simulink model "l5MV"  (R2024a)
settings: Solver=VariableStepAuto  StartTime=0.0  StopTime=200  RelTol=1e-3
settings Model: Creator=sprinkle  LastModifiedBy=ZY395
settings OptimizationCC: ReuseModelBlockBuffer=off
settings RTWCC: GPUComputeCapability=3.5

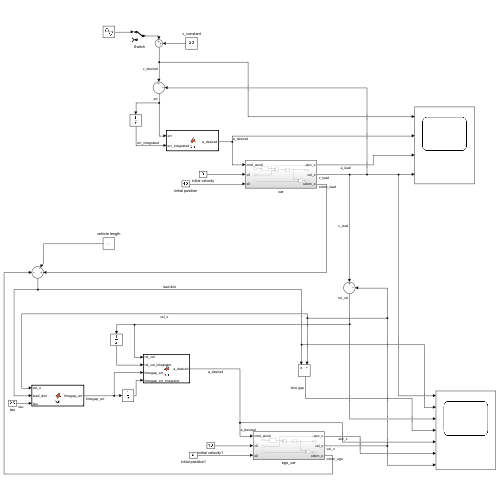
[thumbnail: Simulink's stored preview of the top-level diagram]
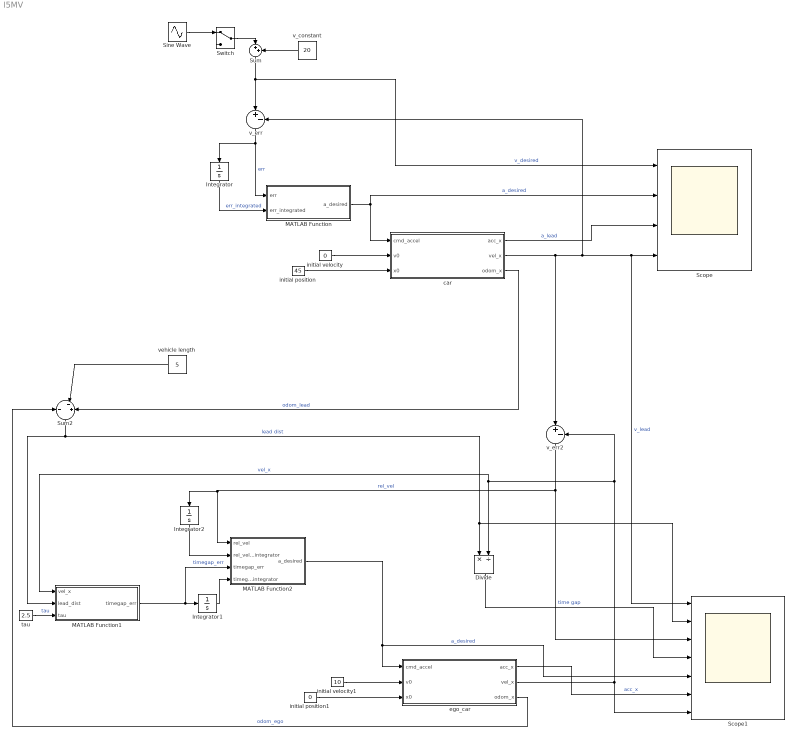
== system l5MV ==
  Divide : Product  Inputs=*/
  Integrator : Integrator
  Integrator1 : Integrator
  Integrator2 : Integrator
  MATLAB Function : MATLAB Function  TreatAsAtomicUnit=on
  MATLAB Function1 : MATLAB Function  TreatAsAtomicUnit=on
  MATLAB Function2 : MATLAB Function  TreatAsAtomicUnit=on
  Scope : Scope  NumInputPorts=4
  Scope1 : Scope  NumInputPorts=7
  Sine Wave : Sin  Amplitude=5  SampleTime=0
  Sum : Sum  Inputs=|++
  Sum2 : Sum  Inputs=-|-+
  Switch : ManualSwitch
  car : Subsystem
  ego_car : Subsystem
  initial position : Constant  Value=45
  initial position1 : Constant  Value=0
  initial velocity : Constant  Value=0
  initial velocity1 : Constant  Value=10
  tau : Constant  Value=2.5
  v_constant : Constant  Value=20
  v_err : Sum  Inputs=|+-
  v_err2 : Sum  Inputs=|+-
  vehicle length : Constant  Value=5
  wires:
  Integrator2/1 -> MATLAB Function2/2(rel_vel_integrator)
  MATLAB Function1/1(timegap_err) -> MATLAB Function2/3(timegap_err), Integrator1/1  "timegap_err"
  ego_car/2(vel_x) -> Scope1/7, Divide/2, MATLAB Function1/1(vel_x), v_err2/2  "vel_x"
  ego_car/1(acc_x) -> Scope1/6  "acc_x"
  MATLAB Function2/1(a_desired) -> ego_car/1(cmd_accel), Scope1/5  "a_desired"
  tau/1 -> MATLAB Function1/3(tau)  "tau"
  v_err2/1 -> Scope1/3, Integrator2/1, MATLAB Function2/1(rel_vel)  "rel_vel"
  MATLAB Function/1(a_desired) -> Scope/2, car/1(cmd_accel)  "a_desired"
  initial velocity1/1 -> ego_car/2(v0)
  ego_car/3(odom_x) -> Sum2/1  "odom_ego"
  Integrator1/1 -> MATLAB Function2/4(timegap_err_integrator)
  Switch/1 -> Sum/1
  vehicle length/1 -> Sum2/2
  Sine Wave/1 -> Switch/1
  Sum/1 -> Scope/1, v_err/1  "v_desired"
  car/3(odom_x) -> Sum2/3  "odom_lead"
  v_constant/1 -> Sum/2
  Sum2/1 -> MATLAB Function1/2(lead_dist), Scope1/2, Divide/1  "lead dist"
  car/2(vel_x) -> v_err/2, Scope1/1, Scope/4, v_err2/1  "v_lead"
  Integrator/1 -> MATLAB Function/2(err_integrated)  "err_integrated"
  Divide/1 -> Scope1/4  "time gap"
  v_err/1 -> MATLAB Function/1(err), Integrator/1  "err"
  initial position/1 -> car/3(x0)
  car/1(acc_x) -> Scope/3  "a_lead"
  initial velocity/1 -> car/2(v0)
  initial position1/1 -> ego_car/3(x0)

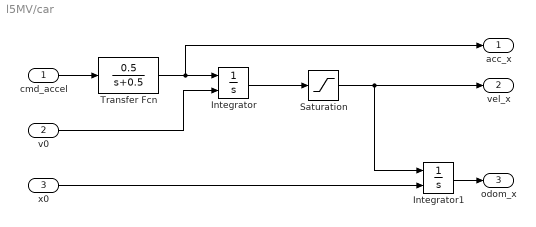
== system l5MV/car ==
  cmd_accel : Inport
  v0 : Inport  Port=2
  x0 : Inport  Port=3
  Integrator : Integrator  InitialConditionSource=external
  Integrator1 : Integrator  InitialConditionSource=external
  Saturation : Saturate  UpperLimit=80  LowerLimit=0
  Transfer Fcn : TransferFcn  Numerator=[0.5]  Denominator=[1 0.5]
  acc_x : Outport
  vel_x : Outport  Port=2
  odom_x : Outport  Port=3
  wires:
  v0/1 -> Integrator/2
  cmd_accel/1 -> Transfer Fcn/1
  Transfer Fcn/1 -> acc_x/1, Integrator/1
  Integrator1/1 -> odom_x/1
  Integrator/1 -> Saturation/1
  x0/1 -> Integrator1/2
  Saturation/1 -> vel_x/1, Integrator1/1

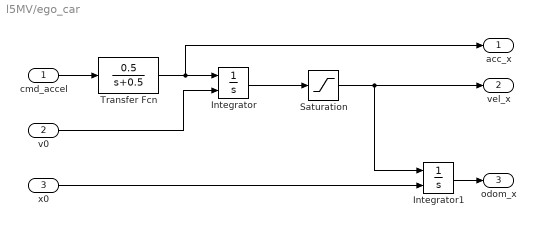
== system l5MV/ego_car ==
  cmd_accel : Inport
  v0 : Inport  Port=2
  x0 : Inport  Port=3
  Integrator : Integrator  InitialConditionSource=external
  Integrator1 : Integrator  InitialConditionSource=external
  Saturation : Saturate  UpperLimit=80  LowerLimit=0
  Transfer Fcn : TransferFcn  Numerator=[0.5]  Denominator=[1 0.5]
  acc_x : Outport
  vel_x : Outport  Port=2
  odom_x : Outport  Port=3
  wires:
  Saturation/1 -> Integrator1/1, vel_x/1
  x0/1 -> Integrator1/2
  Integrator/1 -> Saturation/1
  Integrator1/1 -> odom_x/1
  Transfer Fcn/1 -> Integrator/1, acc_x/1
  cmd_accel/1 -> Transfer Fcn/1
  v0/1 -> Integrator/2

== matlab function l5MV/MATLAB Function1 ==
  data: vel_x input; lead_dist input; tau input; timegap_err output
function timegap_err = fcn(vel_x, lead_dist, tau)

timegap_err = (lead_dist-1)/tau - vel_x; % keep at least 1 meter as safety distance even if both vehicles stop

== matlab function l5MV/MATLAB Function ==
  data: err input; err_integrated input; a_desired output
function a_desired = fcn(err, err_integrated)
a_desired = 0.3*err + 0.01*err_integrated;

if a_desired>1.5
    a_desired=1.5;
elseif a_desired<-3
    a_desired=-3
end;

== matlab function l5MV/MATLAB Function2 ==
  data: rel_vel input; rel_vel_integrator input; a_desired output; timegap_err input; timegap_err_integrator input
function a_desired = fcn(rel_vel, rel_vel_integrator, timegap_err, timegap_err_integrator)
%delt_tau = 0.5;
%tau_max = tau+delt_tau;
%tau_min = tau-delt_tau;
%time_gap = lead_dist/vel_x;

%if time_gap<tau_max && time_gap>tau_min && rel_vel<2
%    ratio = abs(time_gap-timegap_err)/delt_tau;
%    a=a*(exp(ratio)-1)/(exp(1)-1);
%end

alpha1 = 0.8
alpha2 = .5

a = alpha1*rel_vel + alpha2*timegap_err;

%if rel_vel>0 && a<0
%    a = a + 0.001*timegap_err_integrator + 0.001*rel_vel_integrator;
%end

if rel_vel<0 && a>0
    a=0.01*a
end

maxa=1.5;
mina=-3;
a = min(max(mina,a), maxa);


a_desired = a;
